simulink model "EMG_simulation_simulink"  (R2019a)
settings: Solver=VariableStepAuto  StartTime=0.0  StopTime=180  RelTol=1e-3
libraries: dsparch4 x1, simulink x1
settings Model: Creator=patri  LastModifiedBy=patri

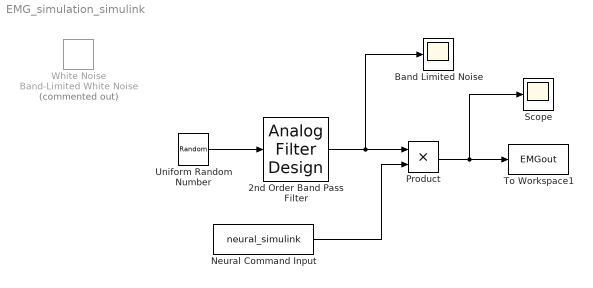
== system EMG_simulation_simulink ==
  2nd Order Band Pass Filter : dsparch4/Analog Filter Design  method=Butterworth  filttype=Bandpass  N=2  Wlo=62.83  Whi=3141.59  Rp=2  Rs=40
  Band Limited Noise : Scope
  Neural Command Input : FromWorkspace  VariableName=neural_simulink  SampleTime=0.001
  Product : Product
  Scope : Scope
  To Workspace1 : ToWorkspace  VariableName=EMGout  SampleTime=0.001
  Uniform Random Number : UniformRandomNumber  Minimum=-6.2e-4  Maximum=6.2e-4  SampleTime=0.001
  White Noise : simulink/Sources/Band-Limited White Noise  Commented=on  Cov=[0.00000000005]  Ts=0.001  seed=[23341]
  wires:
  Neural Command Input/1 -> Product/2
  2nd Order Band Pass Filter/1 -> Product/1, Band Limited Noise/1
  Uniform Random Number/1 -> 2nd Order Band Pass Filter/1
  Product/1 -> Scope/1, To Workspace1/1
